simulink model "gm_sampleModel61706_pp_36_1_sub"  (R2023b)
settings: Solver=VariableStepAuto  StartTime=0.0  StopTime=10.0  RelTol=1e-3
libraries: simulink x39, hdlsllib x2
(part 2 of 2)

== system gm_sampleModel61706_pp_36_1_sub/Subsystem/cfblk38 ==
  emi_179 : Inport  OutDataTypeStr=uint8  PortDimensions=1  SampleTime=1
  Action Port : Inport  Port=2  OutDataTypeStr=boolean  SampleTime=1
  cfblk38 : Signum  SampleTime=1
  cfblk38_out1bypassMux : MultiPortSwitch  DataPortOrder=Zero-based contiguous  Inputs=2  zeroidx=on  OutDataTypeStr=uint8  SampleTime=1  SaturateOnIntegerOverflow=off  InputSameDT=off
  emi_180_bypass : UnitDelay  InitialCondition="fi(0,0,8,0,\"hex\",\"00\")"  SampleTime=1
  emi_180 : Outport  SampleTime=1  InitialOutput=0
  wires:
  Action Port/1 -> cfblk38_out1bypassMux/1
  emi_179/1 -> cfblk38/1
  cfblk38/1 -> cfblk38_out1bypassMux/3
  cfblk38_out1bypassMux/1 -> emi_180_bypass/1, emi_180/1
  emi_180_bypass/1 -> cfblk38_out1bypassMux/2

== system gm_sampleModel61706_pp_36_1_sub/Subsystem/cfblk4 ==
  u : Inport  OutDataTypeStr=double  SampleTime=1
  Compare : RelationalOperator  Operator=<=  OutDataTypeStr=fixdt(0, 8)
  Constant : Constant  DisableCoverage=on  Value=0  OutDataTypeStr=Inherit: Inherit via back propagation  SampleTime=-1  PreserveConstantTs=on
  y : Outport  SampleTime=1
  wires:
  u/1 -> Compare/1
  Compare/1 -> y/1
  Constant/1 -> Compare/2

== system gm_sampleModel61706_pp_36_1_sub/Subsystem/cfblk45_inst ==
  in1 : Inport  OutDataTypeStr=uint8  SampleTime=1
  in2 : Inport  Port=2  OutDataTypeStr=uint8  SampleTime=1
  mul_cfblk45_dotp_mulcomp : Product  Inputs=**  OutDataTypeStr=uint8  SampleTime=1
  out1 : Outport  OutDataTypeStr=uint8  SampleTime=1
  wires:
  in1/1 -> mul_cfblk45_dotp_mulcomp/1
  in2/1 -> mul_cfblk45_dotp_mulcomp/2
  mul_cfblk45_dotp_mulcomp/1 -> out1/1

== system gm_sampleModel61706_pp_36_1_sub/Subsystem/cfblk49 ==
  emi_195 : Inport  OutDataTypeStr=uint8  PortDimensions=1  SampleTime=1
  Action Port : Inport  Port=2  OutDataTypeStr=boolean  SampleTime=1
  cfblk49 : MinMax
  cfblk49_out1bypassMux : MultiPortSwitch  DataPortOrder=Zero-based contiguous  Inputs=2  zeroidx=on  OutDataTypeStr=uint8  SampleTime=1  SaturateOnIntegerOverflow=off  InputSameDT=off
  emi_196_bypass : UnitDelay  InitialCondition="fi(0,0,8,0,\"hex\",\"00\")"  SampleTime=1
  emi_196 : Outport  SampleTime=1  InitialOutput=0
  wires:
  Action Port/1 -> cfblk49_out1bypassMux/1
  emi_195/1 -> cfblk49/1
  cfblk49/1 -> cfblk49_out1bypassMux/3
  cfblk49_out1bypassMux/1 -> emi_196_bypass/1, emi_196/1
  emi_196_bypass/1 -> cfblk49_out1bypassMux/2

== system gm_sampleModel61706_pp_36_1_sub/Subsystem/cfblk5 ==
  u : Inport  OutDataTypeStr=uint8  SampleTime=1
  Compare : RelationalOperator  Operator=<=  OutDataTypeStr=fixdt(0, 8)
  Constant : Constant  DisableCoverage=on  Value=const  OutDataTypeStr=Inherit: Inherit via back propagation  SampleTime=-1
  y : Outport  SampleTime=1
  wires:
  u/1 -> Compare/1
  Compare/1 -> y/1
  Constant/1 -> Compare/2

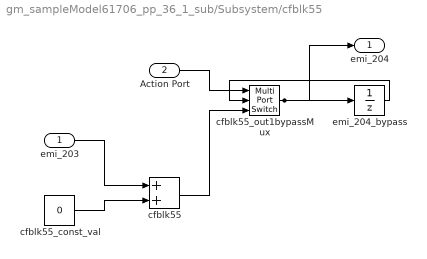
== system gm_sampleModel61706_pp_36_1_sub/Subsystem/cfblk55 ==
  emi_203 : Inport  OutDataTypeStr=uint8  PortDimensions=1  SampleTime=1
  Action Port : Inport  Port=2  OutDataTypeStr=boolean  SampleTime=1
  cfblk55 : Sum  OutDataTypeStr=uint8  AccumDataTypeStr=uint8  RndMeth=Nearest  SampleTime=1
  cfblk55_const_val : Constant  Value=0  VectorParams1D=off  OutDataTypeStr=uint8  SampleTime=1
  cfblk55_out1bypassMux : MultiPortSwitch  DataPortOrder=Zero-based contiguous  Inputs=2  zeroidx=on  OutDataTypeStr=uint8  SampleTime=1  SaturateOnIntegerOverflow=off  InputSameDT=off
  emi_204_bypass : UnitDelay  InitialCondition="fi(0,0,8,0,\"hex\",\"00\")"  SampleTime=1
  emi_204 : Outport  SampleTime=1  InitialOutput=0
  wires:
  Action Port/1 -> cfblk55_out1bypassMux/1
  emi_203/1 -> cfblk55/1
  cfblk55/1 -> cfblk55_out1bypassMux/3
  cfblk55_out1bypassMux/1 -> emi_204_bypass/1, emi_204/1
  emi_204_bypass/1 -> cfblk55_out1bypassMux/2
  cfblk55_const_val/1 -> cfblk55/2

== system gm_sampleModel61706_pp_36_1_sub/Subsystem/cfblk57 ==
  emi_211 : Inport  OutDataTypeStr=uint8  PortDimensions=1  SampleTime=1
  Action Port : Inport  Port=2  OutDataTypeStr=boolean  SampleTime=1
  cfblk57 : Subsystem  mask(Real World Value Increment){}
      mask help: Simulink:masks:RealWorldValueIncrement_MD
      mask Display: disp('V++')
  cfblk57_out1bypassMux : MultiPortSwitch  DataPortOrder=Zero-based contiguous  Inputs=2  zeroidx=on  OutDataTypeStr=uint8  SampleTime=1  SaturateOnIntegerOverflow=off  InputSameDT=off
  emi_212_bypass : UnitDelay  InitialCondition="fi(0,0,8,0,\"hex\",\"00\")"  SampleTime=1
  emi_212 : Outport  SampleTime=1  InitialOutput=0
  wires:
  Action Port/1 -> cfblk57_out1bypassMux/1
  emi_211/1 -> cfblk57/1(u)
  cfblk57/1(y) -> cfblk57_out1bypassMux/3
  cfblk57_out1bypassMux/1 -> emi_212_bypass/1, emi_212/1
  emi_212_bypass/1 -> cfblk57_out1bypassMux/2

== system gm_sampleModel61706_pp_36_1_sub/Subsystem/cfblk60 ==
  u : Inport  OutDataTypeStr=uint8  SampleTime=1
  FixPt Constant : Constant  DisableCoverage=on  OutDataTypeStr=Inherit: Inherit via back propagation  SampleTime=-1
  FixPt Data Type Duplicate : DataTypeDuplicate  DisableCoverage=on  NumInputPorts=3
  FixPt Sum1 : Sum  OutDataTypeStr=Inherit: Inherit via back propagation  InputSameDT=on  LockScale=on
  y : Outport  SampleTime=1
  wires:
  u/1 -> FixPt Sum1/1, FixPt Data Type Duplicate/2
  FixPt Constant/1 -> FixPt Sum1/2, FixPt Data Type Duplicate/3
  FixPt Sum1/1 -> FixPt Data Type Duplicate/1, y/1

== system gm_sampleModel61706_pp_36_1_sub/Subsystem/cfblk64 ==
  emi_147 : Inport  OutDataTypeStr=uint8  PortDimensions=1  SampleTime=1
  Action Port : Inport  Port=2  OutDataTypeStr=boolean  SampleTime=1
  cfblk64 : Gain  Gain="fi(0,0,8,7,\"hex\",\"80\")"  ParamDataTypeStr=fixdt(0, 8, 7)  OutDataTypeStr=fixdt(0, 16, 7)  SampleTime=1
  cfblk64_out1bypassMux : MultiPortSwitch  DataPortOrder=Zero-based contiguous  Inputs=2  zeroidx=on  OutDataTypeStr=fixdt(0, 16, 7)  SampleTime=1  SaturateOnIntegerOverflow=off  InputSameDT=off
  emi_148_bypass : UnitDelay  InitialCondition="fi(0,0,16,7,\"hex\",\"0000\")"  SampleTime=1
  emi_148 : Outport  SampleTime=1  InitialOutput=0
  wires:
  Action Port/1 -> cfblk64_out1bypassMux/1
  emi_147/1 -> cfblk64/1
  cfblk64/1 -> cfblk64_out1bypassMux/3
  cfblk64_out1bypassMux/1 -> emi_148_bypass/1, emi_148/1
  emi_148_bypass/1 -> cfblk64_out1bypassMux/2

== system gm_sampleModel61706_pp_36_1_sub/Subsystem/cfblk66 ==
  emi_227 : Inport  OutDataTypeStr=uint8  PortDimensions=1  SampleTime=1
  Action Port : Inport  Port=2  OutDataTypeStr=boolean  SampleTime=1
  cfblk66 : Sum  Inputs=+
  cfblk66_out1bypassMux : MultiPortSwitch  DataPortOrder=Zero-based contiguous  Inputs=2  zeroidx=on  OutDataTypeStr=uint8  SampleTime=1  SaturateOnIntegerOverflow=off  InputSameDT=off
  emi_228_bypass : UnitDelay  InitialCondition="fi(0,0,8,0,\"hex\",\"00\")"  SampleTime=1
  emi_228 : Outport  SampleTime=1  InitialOutput=0
  wires:
  Action Port/1 -> cfblk66_out1bypassMux/1
  emi_227/1 -> cfblk66/1
  cfblk66/1 -> cfblk66_out1bypassMux/3
  cfblk66_out1bypassMux/1 -> emi_228_bypass/1, emi_228/1
  emi_228_bypass/1 -> cfblk66_out1bypassMux/2

== system gm_sampleModel61706_pp_36_1_sub/Subsystem/cfblk6_inst ==
  in1 : Inport  OutDataTypeStr=uint8  SampleTime=1
  in2 : Inport  Port=2  OutDataTypeStr=uint8  SampleTime=1
  mul_cfblk6_dotp_mulcomp : Product  Inputs=**  OutDataTypeStr=uint8  SampleTime=1
  out1 : Outport  OutDataTypeStr=uint8  SampleTime=1
  wires:
  in1/1 -> mul_cfblk6_dotp_mulcomp/1
  in2/1 -> mul_cfblk6_dotp_mulcomp/2
  mul_cfblk6_dotp_mulcomp/1 -> out1/1

== system gm_sampleModel61706_pp_36_1_sub/Subsystem/cfblk7 ==
  emi_235 : Inport  OutDataTypeStr=uint8  PortDimensions=1  SampleTime=1
  Action Port : Inport  Port=2  OutDataTypeStr=boolean  SampleTime=1
  cfblk7 : MinMax
  cfblk7_out1bypassMux : MultiPortSwitch  DataPortOrder=Zero-based contiguous  Inputs=2  zeroidx=on  OutDataTypeStr=uint8  SampleTime=1  SaturateOnIntegerOverflow=off  InputSameDT=off
  emi_236_bypass : UnitDelay  InitialCondition="fi(0,0,8,0,\"hex\",\"00\")"  SampleTime=1
  emi_236 : Outport  SampleTime=1  InitialOutput=0
  wires:
  Action Port/1 -> cfblk7_out1bypassMux/1
  emi_235/1 -> cfblk7/1
  cfblk7/1 -> cfblk7_out1bypassMux/3
  cfblk7_out1bypassMux/1 -> emi_236_bypass/1, emi_236/1
  emi_236_bypass/1 -> cfblk7_out1bypassMux/2

== system gm_sampleModel61706_pp_36_1_sub/Subsystem/cfblk70 ==
  u : Inport  OutDataTypeStr=uint8  SampleTime=1
  FixPt Constant : Constant  DisableCoverage=on  OutDataTypeStr=Inherit: Inherit via back propagation  SampleTime=-1
  FixPt Data Type Duplicate : DataTypeDuplicate  DisableCoverage=on  NumInputPorts=3
  FixPt Sum1 : Sum  OutDataTypeStr=Inherit: Inherit via back propagation  InputSameDT=on  LockScale=on
  y : Outport  SampleTime=1
  wires:
  u/1 -> FixPt Sum1/1, FixPt Data Type Duplicate/2
  FixPt Constant/1 -> FixPt Sum1/2, FixPt Data Type Duplicate/3
  FixPt Sum1/1 -> FixPt Data Type Duplicate/1, y/1

== system gm_sampleModel61706_pp_36_1_sub/Subsystem/cfblk71_inst ==
  in1 : Inport  OutDataTypeStr=uint8  SampleTime=1
  in2 : Inport  Port=2  OutDataTypeStr=uint8  SampleTime=1
  mul_cfblk71_dotp_mulcomp : Product  Inputs=**  OutDataTypeStr=uint8  SampleTime=1
  out1 : Outport  OutDataTypeStr=uint8  SampleTime=1
  wires:
  in1/1 -> mul_cfblk71_dotp_mulcomp/1
  in2/1 -> mul_cfblk71_dotp_mulcomp/2
  mul_cfblk71_dotp_mulcomp/1 -> out1/1

== system gm_sampleModel61706_pp_36_1_sub/Subsystem/cfblk72 ==
  u : Inport  OutDataTypeStr=double  SampleTime=1
  FixPt Constant : Constant  DisableCoverage=on  OutDataTypeStr=Inherit: Inherit via back propagation  SampleTime=-1
  FixPt Data Type Duplicate : DataTypeDuplicate  DisableCoverage=on  NumInputPorts=3
  FixPt Sum1 : Sum  OutDataTypeStr=Inherit: Inherit via back propagation  InputSameDT=on  LockScale=on
  y : Outport  SampleTime=1
  wires:
  u/1 -> FixPt Sum1/1, FixPt Data Type Duplicate/2
  FixPt Constant/1 -> FixPt Sum1/2, FixPt Data Type Duplicate/3
  FixPt Sum1/1 -> FixPt Data Type Duplicate/1, y/1

== system gm_sampleModel61706_pp_36_1_sub/Subsystem/cfblk74 ==
  emi_243 : Inport  OutDataTypeStr=fixdt(0, 16, 7)  PortDimensions=1  SampleTime=1
  Action Port : Inport  Port=2  OutDataTypeStr=boolean  SampleTime=1
  Reshape : Reshape
  cfblk74_out1bypassMux : MultiPortSwitch  DataPortOrder=Zero-based contiguous  Inputs=2  zeroidx=on  OutDataTypeStr=fixdt(0, 16, 7)  SampleTime=1  SaturateOnIntegerOverflow=off  InputSameDT=off
  emi_244_bypass : UnitDelay  InitialCondition="fi(0,0,16,7,\"hex\",\"0000\")"  SampleTime=1
  emi_244 : Outport  SampleTime=1  InitialOutput=0
  wires:
  Action Port/1 -> cfblk74_out1bypassMux/1
  emi_243/1 -> Reshape/1
  Reshape/1 -> cfblk74_out1bypassMux/3
  cfblk74_out1bypassMux/1 -> emi_244_bypass/1, emi_244/1
  emi_244_bypass/1 -> cfblk74_out1bypassMux/2

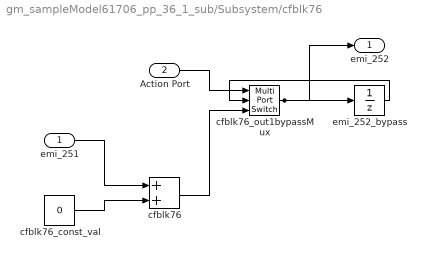
== system gm_sampleModel61706_pp_36_1_sub/Subsystem/cfblk76 ==
  emi_251 : Inport  OutDataTypeStr=uint8  PortDimensions=1  SampleTime=1
  Action Port : Inport  Port=2  OutDataTypeStr=boolean  SampleTime=1
  cfblk76 : Sum  OutDataTypeStr=uint8  AccumDataTypeStr=uint8  RndMeth=Nearest  SampleTime=1
  cfblk76_const_val : Constant  Value=0  VectorParams1D=off  OutDataTypeStr=uint8  SampleTime=1
  cfblk76_out1bypassMux : MultiPortSwitch  DataPortOrder=Zero-based contiguous  Inputs=2  zeroidx=on  OutDataTypeStr=uint8  SampleTime=1  SaturateOnIntegerOverflow=off  InputSameDT=off
  emi_252_bypass : UnitDelay  InitialCondition="fi(0,0,8,0,\"hex\",\"00\")"  SampleTime=1
  emi_252 : Outport  SampleTime=1  InitialOutput=0
  wires:
  Action Port/1 -> cfblk76_out1bypassMux/1
  emi_251/1 -> cfblk76/1
  cfblk76/1 -> cfblk76_out1bypassMux/3
  cfblk76_out1bypassMux/1 -> emi_252_bypass/1, emi_252/1
  emi_252_bypass/1 -> cfblk76_out1bypassMux/2
  cfblk76_const_val/1 -> cfblk76/2

== system gm_sampleModel61706_pp_36_1_sub/Subsystem/cfblk8 ==
  emi_259 : Inport  OutDataTypeStr=uint8  PortDimensions=1  SampleTime=1
  Action Port : Inport  Port=2  OutDataTypeStr=boolean  SampleTime=1
  cfblk8 : Abs  SampleTime=1  OutDataTypeStr=uint8  SaturateOnIntegerOverflow=off
  cfblk8_out1bypassMux : MultiPortSwitch  DataPortOrder=Zero-based contiguous  Inputs=2  zeroidx=on  OutDataTypeStr=uint8  SampleTime=1  SaturateOnIntegerOverflow=off  InputSameDT=off
  emi_260_bypass : UnitDelay  InitialCondition="fi(0,0,8,0,\"hex\",\"00\")"  SampleTime=1
  emi_260 : Outport  SampleTime=1  InitialOutput=0
  wires:
  Action Port/1 -> cfblk8_out1bypassMux/1
  emi_259/1 -> cfblk8/1
  cfblk8/1 -> cfblk8_out1bypassMux/3
  cfblk8_out1bypassMux/1 -> emi_260_bypass/1, emi_260/1
  emi_260_bypass/1 -> cfblk8_out1bypassMux/2

== system gm_sampleModel61706_pp_36_1_sub/Subsystem/cfblk80 ==
  u : Inport  OutDataTypeStr=uint8  SampleTime=1
  FixPt Constant : Constant  DisableCoverage=on  OutDataTypeStr=Inherit: Inherit via back propagation  SampleTime=-1
  FixPt Data Type Duplicate : DataTypeDuplicate  DisableCoverage=on  NumInputPorts=3
  FixPt Sum1 : Sum  OutDataTypeStr=Inherit: Inherit via back propagation  InputSameDT=on  LockScale=on
  y : Outport  SampleTime=1
  wires:
  u/1 -> FixPt Sum1/1, FixPt Data Type Duplicate/2
  FixPt Constant/1 -> FixPt Sum1/2, FixPt Data Type Duplicate/3
  FixPt Sum1/1 -> FixPt Data Type Duplicate/1, y/1

== system gm_sampleModel61706_pp_36_1_sub/Subsystem/cfblk81 ==
  u : Inport  OutDataTypeStr=uint8  SampleTime=1
  FixPt Constant : Constant  DisableCoverage=on  OutDataTypeStr=Inherit: Inherit via back propagation  SampleTime=-1
  FixPt Data Type Duplicate : DataTypeDuplicate  DisableCoverage=on  NumInputPorts=3
  FixPt Sum1 : Sum  OutDataTypeStr=Inherit: Inherit via back propagation  InputSameDT=on  LockScale=on
  y : Outport  SampleTime=1
  wires:
  u/1 -> FixPt Sum1/1, FixPt Data Type Duplicate/2
  FixPt Constant/1 -> FixPt Sum1/2, FixPt Data Type Duplicate/3
  FixPt Sum1/1 -> FixPt Data Type Duplicate/1, y/1

== system gm_sampleModel61706_pp_36_1_sub/Subsystem/cfblk86_inst ==
  in1 : Inport  OutDataTypeStr=uint8  SampleTime=1
  in2 : Inport  Port=2  OutDataTypeStr=uint8  SampleTime=1
  mul_cfblk86_dotp_mulcomp : Product  Inputs=**  OutDataTypeStr=uint8  SampleTime=1
  out1 : Outport  OutDataTypeStr=uint8  SampleTime=1
  wires:
  in1/1 -> mul_cfblk86_dotp_mulcomp/1
  in2/1 -> mul_cfblk86_dotp_mulcomp/2
  mul_cfblk86_dotp_mulcomp/1 -> out1/1

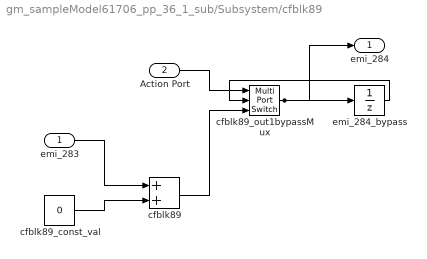
== system gm_sampleModel61706_pp_36_1_sub/Subsystem/cfblk89 ==
  emi_283 : Inport  OutDataTypeStr=uint8  PortDimensions=1  SampleTime=1
  Action Port : Inport  Port=2  OutDataTypeStr=boolean  SampleTime=1
  cfblk89 : Sum  OutDataTypeStr=uint8  AccumDataTypeStr=uint8  RndMeth=Nearest  SampleTime=1
  cfblk89_const_val : Constant  Value=0  VectorParams1D=off  OutDataTypeStr=uint8  SampleTime=1
  cfblk89_out1bypassMux : MultiPortSwitch  DataPortOrder=Zero-based contiguous  Inputs=2  zeroidx=on  OutDataTypeStr=uint8  SampleTime=1  SaturateOnIntegerOverflow=off  InputSameDT=off
  emi_284_bypass : UnitDelay  InitialCondition="fi(0,0,8,0,\"hex\",\"00\")"  SampleTime=1
  emi_284 : Outport  SampleTime=1  InitialOutput=0
  wires:
  Action Port/1 -> cfblk89_out1bypassMux/1
  emi_283/1 -> cfblk89/1
  cfblk89/1 -> cfblk89_out1bypassMux/3
  cfblk89_out1bypassMux/1 -> emi_284_bypass/1, emi_284/1
  emi_284_bypass/1 -> cfblk89_out1bypassMux/2
  cfblk89_const_val/1 -> cfblk89/2

== system gm_sampleModel61706_pp_36_1_sub/Subsystem/cfblk9 ==
  u : Inport  OutDataTypeStr=uint8  SampleTime=1
  FixPt Constant : Constant  DisableCoverage=on  OutDataTypeStr=Inherit: Inherit via back propagation  SampleTime=-1
  FixPt Data Type Duplicate : DataTypeDuplicate  DisableCoverage=on  NumInputPorts=3
  FixPt Sum1 : Sum  OutDataTypeStr=Inherit: Inherit via back propagation  InputSameDT=on  LockScale=on
  y : Outport  SampleTime=1
  wires:
  u/1 -> FixPt Sum1/1, FixPt Data Type Duplicate/2
  FixPt Constant/1 -> FixPt Sum1/2, FixPt Data Type Duplicate/3
  FixPt Sum1/1 -> FixPt Data Type Duplicate/1, y/1

== system gm_sampleModel61706_pp_36_1_sub/Subsystem/cfblk96 ==
  emi_291 : Inport  OutDataTypeStr=uint8  PortDimensions=1  SampleTime=1
  Action Port : Inport  Port=2  OutDataTypeStr=boolean  SampleTime=1
  cfblk96 : Signum  SampleTime=1
  cfblk96_out1bypassMux : MultiPortSwitch  DataPortOrder=Zero-based contiguous  Inputs=2  zeroidx=on  OutDataTypeStr=uint8  SampleTime=1  SaturateOnIntegerOverflow=off  InputSameDT=off
  emi_292_bypass : UnitDelay  InitialCondition="fi(0,0,8,0,\"hex\",\"00\")"  SampleTime=1
  emi_292 : Outport  SampleTime=1  InitialOutput=0
  wires:
  Action Port/1 -> cfblk96_out1bypassMux/1
  emi_291/1 -> cfblk96/1
  cfblk96/1 -> cfblk96_out1bypassMux/3
  cfblk96_out1bypassMux/1 -> emi_292_bypass/1, emi_292/1
  emi_292_bypass/1 -> cfblk96_out1bypassMux/2

== system gm_sampleModel61706_pp_36_1_sub/Subsystem/cfblk97_inst ==
  in1 : Inport  OutDataTypeStr=uint8  SampleTime=1
  in2 : Inport  Port=2  OutDataTypeStr=uint8  SampleTime=1
  mul_cfblk97_dotp_mulcomp : Product  Inputs=**  OutDataTypeStr=uint8  SampleTime=1
  out1 : Outport  OutDataTypeStr=uint8  SampleTime=1
  wires:
  in1/1 -> mul_cfblk97_dotp_mulcomp/1
  in2/1 -> mul_cfblk97_dotp_mulcomp/2
  mul_cfblk97_dotp_mulcomp/1 -> out1/1

== system gm_sampleModel61706_pp_36_1_sub/Subsystem/cfblk98 ==
  emi_299 : Inport  OutDataTypeStr=uint8  PortDimensions=1  SampleTime=1
  Action Port : Inport  Port=2  OutDataTypeStr=boolean  SampleTime=1
  cfblk98 : Gain  Gain="fi(0,0,8,7,\"hex\",\"80\")"  ParamDataTypeStr=fixdt(0, 8, 7)  OutDataTypeStr=fixdt(0, 16, 7)  SampleTime=1
  cfblk98_out1bypassMux : MultiPortSwitch  DataPortOrder=Zero-based contiguous  Inputs=2  zeroidx=on  OutDataTypeStr=fixdt(0, 16, 7)  SampleTime=1  SaturateOnIntegerOverflow=off  InputSameDT=off
  emi_300_bypass : UnitDelay  InitialCondition="fi(0,0,16,7,\"hex\",\"0000\")"  SampleTime=1
  emi_300 : Outport  SampleTime=1  InitialOutput=0
  wires:
  Action Port/1 -> cfblk98_out1bypassMux/1
  emi_299/1 -> cfblk98/1
  cfblk98/1 -> cfblk98_out1bypassMux/3
  cfblk98_out1bypassMux/1 -> emi_300_bypass/1, emi_300/1
  emi_300_bypass/1 -> cfblk98_out1bypassMux/2

== system gm_sampleModel61706_pp_36_1_sub/Subsystem/cfblk99 ==
  emi_307 : Inport  OutDataTypeStr=uint8  PortDimensions=1  SampleTime=1
  Action Port : Inport  Port=2  OutDataTypeStr=boolean  SampleTime=1
  Reshape : Reshape
  cfblk99_out1bypassMux : MultiPortSwitch  DataPortOrder=Zero-based contiguous  Inputs=2  zeroidx=on  OutDataTypeStr=uint8  SampleTime=1  SaturateOnIntegerOverflow=off  InputSameDT=off
  emi_308_bypass : UnitDelay  InitialCondition="fi(0,0,8,0,\"hex\",\"00\")"  SampleTime=1
  emi_308 : Outport  SampleTime=1  InitialOutput=0
  wires:
  Action Port/1 -> cfblk99_out1bypassMux/1
  emi_307/1 -> Reshape/1
  Reshape/1 -> cfblk99_out1bypassMux/3
  cfblk99_out1bypassMux/1 -> emi_308_bypass/1, emi_308/1
  emi_308_bypass/1 -> cfblk99_out1bypassMux/2

== system gm_sampleModel61706_pp_36_1_sub/Subsystem/cfblk197/cfblk197 ==
  in0 : Inport  OutDataTypeStr=uint8  SampleTime=1
  Action Port_out2 : EnablePort  OutDataTypeStr=boolean
  cfblk197 : Delay  DelayLength=double(2)  InitialCondition=0
  out0 : Outport  OutDataTypeStr=uint8  SampleTime=1  InitialOutput=0
  wires:
  cfblk197/1 -> out0/1
  in0/1 -> cfblk197/1

== system gm_sampleModel61706_pp_36_1_sub/Subsystem/cfblk200/cfblk200 ==
  in0 : Inport  OutDataTypeStr=uint8  SampleTime=1
  Action Port_out2 : EnablePort  OutDataTypeStr=boolean
  cfblk200 : Delay  DelayLength=double(2)  InitialCondition=0
  out0 : Outport  OutDataTypeStr=uint8  SampleTime=1  InitialOutput=0
  wires:
  cfblk200/1 -> out0/1
  in0/1 -> cfblk200/1

== system gm_sampleModel61706_pp_36_1_sub/Subsystem/cfblk28/cfblk28 ==
  u : Inport  OutDataTypeStr=uint8  SampleTime=1
  FixPt Constant : Constant  DisableCoverage=on  OutDataTypeStr=Inherit: Inherit via back propagation  SampleTime=-1
  FixPt Data Type Duplicate : DataTypeDuplicate  DisableCoverage=on  NumInputPorts=3
  FixPt Sum1 : Sum  OutDataTypeStr=Inherit: Inherit via back propagation  InputSameDT=on  LockScale=on
  y : Outport  SampleTime=1  InitialOutput=0
  wires:
  u/1 -> FixPt Sum1/1, FixPt Data Type Duplicate/2
  FixPt Constant/1 -> FixPt Sum1/2, FixPt Data Type Duplicate/3
  FixPt Sum1/1 -> FixPt Data Type Duplicate/1, y/1

== system gm_sampleModel61706_pp_36_1_sub/Subsystem/cfblk37/cfblk37 ==
  u : Inport  OutDataTypeStr=uint8  SampleTime=1
  FixPt Constant : Constant  DisableCoverage=on  OutDataTypeStr=Inherit: Inherit via back propagation  SampleTime=-1
  FixPt Data Type Duplicate : DataTypeDuplicate  DisableCoverage=on  NumInputPorts=3
  FixPt Sum1 : Sum  OutDataTypeStr=Inherit: Inherit via back propagation  InputSameDT=on  LockScale=on
  y : Outport  SampleTime=1  InitialOutput=0
  wires:
  u/1 -> FixPt Sum1/1, FixPt Data Type Duplicate/2
  FixPt Constant/1 -> FixPt Sum1/2, FixPt Data Type Duplicate/3
  FixPt Sum1/1 -> FixPt Data Type Duplicate/1, y/1

== system gm_sampleModel61706_pp_36_1_sub/Subsystem/cfblk57/cfblk57 ==
  u : Inport  OutDataTypeStr=uint8  SampleTime=1
  FixPt Constant : Constant  DisableCoverage=on  OutDataTypeStr=Inherit: Inherit via back propagation  SampleTime=-1
  FixPt Data Type Duplicate : DataTypeDuplicate  DisableCoverage=on  NumInputPorts=3
  FixPt Sum1 : Sum  OutDataTypeStr=Inherit: Inherit via back propagation  InputSameDT=on  LockScale=on
  y : Outport  SampleTime=1  InitialOutput=0
  wires:
  u/1 -> FixPt Sum1/1, FixPt Data Type Duplicate/2
  FixPt Constant/1 -> FixPt Sum1/2, FixPt Data Type Duplicate/3
  FixPt Sum1/1 -> FixPt Data Type Duplicate/1, y/1
